simulink model "rover_control"  (R2019b)
settings: Solver=ode3  StartTime=0.0  StopTime=inf  RelTol=1e-3  EnableMultiTasking=on
undefined symbols (not defined in the file or in its folder): Discrete, Time
libraries: embdlinuxlib x13, simulink x3, ctrlSharedLib x2, raspberrypilib x2, sensehatlib x1
(part 2 of 2)

== system rover_control/Plant/Subsystem1/Subsystem1/RGB1 ==
  In1 : Inport
  In2 : Inport  Port=2
  In3 : Inport  Port=3
  B1 : embdlinuxlib/GPIO Write  board=Pi 3 Model B+  gpio=24  direction=Output  blockPlatform=Raspberry Pi
      settings: SourceProductName=Simulink Support Package for Raspberry Pi Hardware  SourceProductBaseCode=RASPPI
  G1 : embdlinuxlib/GPIO Write  board=Pi 3 Model B+  gpio=23  direction=Output  blockPlatform=Raspberry Pi
      settings: SourceProductName=Simulink Support Package for Raspberry Pi Hardware  SourceProductBaseCode=RASPPI
  R1 : embdlinuxlib/GPIO Write  board=Pi 3 Model B+  gpio=22  direction=Output  blockPlatform=Raspberry Pi
      settings: SourceProductName=Simulink Support Package for Raspberry Pi Hardware  SourceProductBaseCode=RASPPI
  wires:
  In1/1 -> R1/1
  In3/1 -> B1/1
  In2/1 -> G1/1

== system rover_control/Plant/Subsystem1/Subsystem1/RGB2 ==
  In1 : Inport
  In2 : Inport  Port=2
  In3 : Inport  Port=3
  B1 : embdlinuxlib/GPIO Write  board=Model B+  gpio=25  direction=Output  blockPlatform=Raspberry Pi
      settings: SourceProductName=Simulink Support Package for Raspberry Pi Hardware  SourceProductBaseCode=RASPPI
  G1 : embdlinuxlib/GPIO Write  board=Model B+  gpio=9  direction=Output  blockPlatform=Raspberry Pi
      settings: SourceProductName=Simulink Support Package for Raspberry Pi Hardware  SourceProductBaseCode=RASPPI
  R1 : embdlinuxlib/GPIO Write  board=Model B+  gpio=10  direction=Output  blockPlatform=Raspberry Pi
      settings: SourceProductName=Simulink Support Package for Raspberry Pi Hardware  SourceProductBaseCode=RASPPI
  wires:
  In2/1 -> G1/1
  In3/1 -> B1/1
  In1/1 -> R1/1

== system rover_control/Plant/Subsystem1/Subsystem1/ServoControl ==
  cam_ud : Inport
  cam_lr : Inport  Port=2
  whl_lr : Inport  Port=3
  Ground : Ground
  MATLAB System : MATLABSystem  System=PCA9685  SlaveAddress=hex2dec('40')  Frequency=60
      mask Type: PCA9685
      mask Display:
      | disp('PCA9685');
      | port_label('input',1,'u1');
      | port_label('input',2,'u2');
      | port_label('input',3,'u3');
      | port_label('input',4,'u4');
      | port_label('input',5,'u5');
      | port_label('input',6,'u6');
      | port_label('input',7,'u7');
      | port_label('input',8,'u8');
      | port_label('input',9,'u9');
      | port_label('input',10,'u10');
      | port_label('input',11,'u11');
      | port_label('input',12,'u12');
  wires:
  Ground/1 -> MATLAB System/11, MATLAB System/12, MATLAB System/10, MATLAB System/4, MATLAB System/5, MATLAB System/6, MATLAB System/7, MATLAB System/8, MATLAB System/9
  cam_lr/1 -> MATLAB System/2
  whl_lr/1 -> MATLAB System/3
  cam_ud/1 -> MATLAB System/1

== system rover_control/Plant/Subsystem2/RPiSystem/RPiSerialSource ==
  Compare To Constant : simulink/Logic and Bit Operations/Compare To Constant  relop===  const=uint8(0)  OutDataTypeStr=boolean
  Constant1 : Constant  Value=zeros(1,164)  OutDataTypeStr=uint8
  Serial Read : raspberrypilib/Serial Read  board=Pi 3 Model B  SCIModule_=/dev/ttyS0  Baudrate_=9600  Parity=None  StopBits_=1  HardwareFlowControl=None  ByteOrder=LittleEndian  DataLength=164  DataType=uint8  OutputStatus=on  SampleTime=0.1  blockPlatform=RaspberryPi
      settings: SourceProductName=Simulink Support Package for Raspberry Pi Hardware  SourceProductBaseCode=RASPPI
  Switch : Switch  Criteria=u2 > Threshold
  gps_vector : Outport
  wires:
  Switch/1 -> gps_vector/1  "gps_vector"
  Serial Read/2 -> Compare To Constant/1
  Constant1/1 -> Switch/3
  Serial Read/1 -> Switch/1  "gps_vector"
  Compare To Constant/1 -> Switch/2

== system rover_control/Plant/Subsystem2/RPiSystem/Tracking3CH ==
  Bus Creator : BusCreator  Inputs=3
  C : embdlinuxlib/GPIO Read  board=Pi 3 Model B+  gpio=16  internalResistor=Off  sampleTime=0.1  direction=Input  blockPlatform=Raspberry Pi
      settings: SourceProductName=Simulink Support Package for Raspberry Pi Hardware  SourceProductBaseCode=RASPPI
  Display : Display
  Display1 : Display
  Display2 : Display
  L : embdlinuxlib/GPIO Read  board=Pi 3 Model B+  gpio=19  internalResistor=Off  sampleTime=0.1  direction=Input  blockPlatform=Raspberry Pi
      settings: SourceProductName=Simulink Support Package for Raspberry Pi Hardware  SourceProductBaseCode=RASPPI
  NOT : Logic  Operator=NOT  IconShape=distinctive  AllPortsSameDT=off  OutDataTypeStr=boolean
  NOT1 : Logic  Operator=NOT  IconShape=distinctive  AllPortsSameDT=off  OutDataTypeStr=boolean
  NOT2 : Logic  Operator=NOT  IconShape=distinctive  AllPortsSameDT=off  OutDataTypeStr=boolean
  R : embdlinuxlib/GPIO Read  board=Pi 3 Model B+  gpio=20  internalResistor=Off  sampleTime=0.1  direction=Input  blockPlatform=Raspberry Pi
      settings: SourceProductName=Simulink Support Package for Raspberry Pi Hardware  SourceProductBaseCode=RASPPI
  tracking : Outport
  wires:
  Bus Creator/1 -> tracking/1
  L/1 -> NOT/1
  C/1 -> NOT1/1
  R/1 -> NOT2/1
  NOT/1 -> Display/1, Bus Creator/1  "leftLineDetected"
  NOT1/1 -> Display1/1, Bus Creator/2  "centerLineDetected"
  NOT2/1 -> Display2/1, Bus Creator/3  "rightLineDetected"

== system rover_control/Plant/Subsystem2/RPiSystem/UltrasonicSensor ==
  MATLAB System : MATLABSystem  System=UltrasonicRead  EchoPinNumber=echo_gpio  TriggerPinNumber=trigger_gpio  SampleTime=sampleTime
      mask Type: UltrasonicRead
      mask Display:
      | disp('Ultrasonic Read');
      | port_label('output',1,'y');
  Out1 : Outport  VectorParamsAs1DForOutWhenUnconnected=off
  wires:
  MATLAB System/1 -> Out1/1

== system rover_control/Controller/Subsystem/GPS/CharacterBufferLoad/NMEASentenceExtract ==
  serial_vector : Inport
  ASCII to String : ASCIIToString
  MATLAB Function : MATLAB Function  TreatAsAtomicUnit=on
  string : Outport
  wires:
  serial_vector/1 -> MATLAB Function/1(u)
  ASCII to String/1 -> string/1
  MATLAB Function/1(y) -> ASCII to String/1

== system rover_control/Controller/Subsystem/GPS/GGA Decoder/Subsystem ==
  In1 : Inport
  Constant : Constant  OutDataTypeStr=uint8
  Constant1 : Constant  Value=2  OutDataTypeStr=uint8
  Constant2 : Constant  Value=3  OutDataTypeStr=uint8
  Constant4 : Constant  Value=5  OutDataTypeStr=uint8
  String Concatenate : StringConcatenate  Inputs=5
  String Constant : StringConstant  String="\":\""
  Substring : Substring
  Substring1 : Substring
  Substring2 : Substring
  Out1 : Outport  VectorParamsAs1DForOutWhenUnconnected=off
  wires:
  Constant/1 -> Substring/2
  Constant2/1 -> Substring1/2
  Constant4/1 -> Substring2/2
  In1/1 -> Substring2/1, Substring/1, Substring1/1
  Constant1/1 -> Substring2/3, Substring1/3, Substring/3
  Substring1/1 -> String Concatenate/3
  Substring/1 -> String Concatenate/1
  Substring2/1 -> String Concatenate/5
  String Constant/1 -> String Concatenate/4, String Concatenate/2
  String Concatenate/1 -> Out1/1

== system rover_control/Controller/Subsystem/GPS/GLL Decoder/Subsystem ==
  In1 : Inport
  Constant : Constant  OutDataTypeStr=uint8
  Constant1 : Constant  Value=2  OutDataTypeStr=uint8
  Constant2 : Constant  Value=3  OutDataTypeStr=uint8
  Constant4 : Constant  Value=5  OutDataTypeStr=uint8
  String Concatenate : StringConcatenate  Inputs=5
  String Constant : StringConstant  String="\":\""
  Substring : Substring
  Substring1 : Substring
  Substring2 : Substring
  Out1 : Outport  VectorParamsAs1DForOutWhenUnconnected=off
  wires:
  String Concatenate/1 -> Out1/1
  String Constant/1 -> String Concatenate/2, String Concatenate/4
  Substring2/1 -> String Concatenate/5
  Substring/1 -> String Concatenate/1
  Substring1/1 -> String Concatenate/3
  Constant1/1 -> Substring/3, Substring1/3, Substring2/3
  In1/1 -> Substring1/1, Substring/1, Substring2/1
  Constant4/1 -> Substring2/2
  Constant2/1 -> Substring1/2
  Constant/1 -> Substring/2

== system rover_control/Controller/Subsystem/GPS/GSA Decoder/Subsystem ==
  In1 : Inport
  ASCII to String : ASCIIToString
  ASCII to String1 : ASCIIToString
  MATLAB Function : MATLAB Function  TreatAsAtomicUnit=on
  Scan String : ScanString  Format="\"%hu,%hu,%hu,%hu,%hu,%hu,%hu,%hu,%hu,%hu,%hu,%hu\""
  String to ASCII : StringToASCII  OutputVectorSize=80
  Vector Concatenate : Concatenate  NumInputs=12
  prns : Outport
  rem : Outport  Port=2
  wires:
  In1/1 -> String to ASCII/1
  String to ASCII/1 -> MATLAB Function/1(u)
  MATLAB Function/2(prns) -> ASCII to String1/1
  MATLAB Function/1(y) -> ASCII to String/1
  ASCII to String/1 -> rem/1
  ASCII to String1/1 -> Scan String/1
  Scan String/1 -> Vector Concatenate/1
  Scan String/2 -> Vector Concatenate/2
  Scan String/3 -> Vector Concatenate/3
  Scan String/4 -> Vector Concatenate/4
  Scan String/5 -> Vector Concatenate/5
  Scan String/6 -> Vector Concatenate/6
  Scan String/7 -> Vector Concatenate/7
  Scan String/8 -> Vector Concatenate/8
  Scan String/9 -> Vector Concatenate/9
  Scan String/10 -> Vector Concatenate/10
  Scan String/11 -> Vector Concatenate/11
  Scan String/12 -> Vector Concatenate/12
  Vector Concatenate/1 -> prns/1

== system rover_control/Controller/Subsystem/GPS/RMC Decoder/Subsystem ==
  In1 : Inport
  Constant : Constant  OutDataTypeStr=uint8
  Constant1 : Constant  Value=2  OutDataTypeStr=uint8
  Constant2 : Constant  Value=3  OutDataTypeStr=uint8
  Constant4 : Constant  Value=5  OutDataTypeStr=uint8
  String Concatenate : StringConcatenate  Inputs=5
  String Constant : StringConstant  String="\":\""
  Substring : Substring
  Substring1 : Substring
  Substring2 : Substring
  Out1 : Outport  VectorParamsAs1DForOutWhenUnconnected=off
  wires:
  Constant/1 -> Substring/2
  Constant2/1 -> Substring1/2
  Constant4/1 -> Substring2/2
  In1/1 -> Substring2/1, Substring/1, Substring1/1
  Constant1/1 -> Substring2/3, Substring1/3, Substring/3
  Substring1/1 -> String Concatenate/3
  Substring/1 -> String Concatenate/1
  Substring2/1 -> String Concatenate/5
  String Constant/1 -> String Concatenate/4, String Concatenate/2
  String Concatenate/1 -> Out1/1

== system rover_control/Controller/Subsystem/GPS/RMC Decoder/Subsystem1 ==
  In1 : Inport
  Constant : Constant  Value=3  OutDataTypeStr=uint8
  Constant1 : Constant  Value=2  OutDataTypeStr=uint8
  Constant2 : Constant  OutDataTypeStr=uint8
  Constant4 : Constant  Value=5  OutDataTypeStr=uint8
  String Concatenate : StringConcatenate  Inputs=5
  String Constant : StringConstant  String="\"/\""
  Substring : Substring
  Substring1 : Substring
  Substring2 : Substring
  Out1 : Outport  VectorParamsAs1DForOutWhenUnconnected=off
  wires:
  Constant/1 -> Substring/2
  Constant2/1 -> Substring1/2
  Constant4/1 -> Substring2/2
  In1/1 -> Substring2/1, Substring/1, Substring1/1
  Constant1/1 -> Substring2/3, Substring1/3, Substring/3
  Substring1/1 -> String Concatenate/3
  Substring/1 -> String Concatenate/1
  Substring2/1 -> String Concatenate/5
  String Constant/1 -> String Concatenate/4, String Concatenate/2
  String Concatenate/1 -> Out1/1

== matlab function rover_control/Controller/Subsystem/GPS/GSA Decoder/Subsystem/MATLAB Function ==
  data: y output; u input; prns output
function [y, prns] = gsa(u)
%UNTITLED Summary of this function goes here
%   Detailed explanation goes here
y = zeros(size(u),'uint8');
num_prns = 12;
prns = zeros(size(u),'uint8');
idx = find(u == hex2dec('2c')) ;
% prns = zeros(1,12,'uint16');
%A,3,66,84,74,75,76,85,,,,,,,1.47,0.78,1.24,*17

sIdx = 1;
% for i = 1:length(prns)
%     new_string = u(sIdx:idx(i)-1);
%     if (~isempty(new_string))
%         prns(i) = uint16(str2double(new_string));
%     end
%     sIdx = idx(i)+1;
% end
for i=1:num_prns
    %66,34,23,53,,,,,,,,,,
    new_string = u(sIdx:idx(i)-1);
    if (~isempty(new_string))
        prns(sIdx:sIdx+length(new_string)) = [new_string, ','];
        z = length(new_string);
    else
        if (i == num_prns)
            prns(sIdx) = '0';
            z = 1;
        else
            prns(sIdx:sIdx+1) = '0,';
            z = 1;
        end
    end
%     prns(pIdx:idx(i)) = u(sIdx:idx(i));
    sIdx = sIdx + z + 1;
%     disp(i)
%     disp(char(prns))
end
y(1:length(u)-idx(12)) = u(idx(12)+1:end);
% pdop = str2double(char(u(sIdx:
% hdop = 
% vdop = 
% checksum = 
end
% function [y, prns] = gsa_u(u)
% y = zeros(1,80,'uint8');
% [z,prns] = gsa(u);
% y(1:length(z)) = z;
% end

== matlab function rover_control/Controller/Subsystem/GPS/CharacterBufferLoad/NMEASentenceExtract/MATLAB Function ==
  data: u input; y output size=[1 80]
function y  = gps_data_handle(u)
persistent start;
persistent new_input;
persistent prev_u;
% \r - 0xD (carriage return) \n - 0xA )(line feed)
% 
% d = find(u == hex2dec('d'));
% r = find(u == hex2dec('a'));
%
% $ - decimal 36 hex 0x24
if (isempty(start))
    start = false;
    new_input = zeros(1,length(u)*2,'like',u);
    prev_u = zeros(size(u),'like',u);
end
if (~start)
    start = true;
    prev_u = u;
    % check if data is complete
    if (u(1) ~= hex2dec('24'))
        % find first index that has '$'
        idx = find(u,1,'first');
%         z = zeros(size(u));
        u = shift_vector(u, idx(1)-1);
    end
    new_input(1:length(u)) = u;
end
        
if (~isequal(u,prev_u))
    idx = find(new_input == 0,1,'first');
    new_input(idx(1):idx(1)+length(u)-1) = u(1:end);
    prev_u = u;
end

sentence = zeros(1,80, 'like',u);
idx = find(new_input == hex2dec('24'), 2, 'first');
if (length(idx) == 2)
    % this is needed if the carriage return and line feed get treated as
    % separate characters like it does in raspberry pi serial block
    crlf = 2;
    sentence(1:idx(2)-idx(1)-crlf) = new_input(idx(1):idx(2)-1-crlf);
    new_input = shift_vector(new_input, idx(2)-1);
end

y = sentence;
end

function y = shift_vector(u, K)
 
y=zeros(size(u),'like',u);
% n=2; %Shift units
y(1:end-K+1)=u(K:end);
end

== matlab function rover_control/Controller/Subsystem/GPS/VTG Decoder/MATLAB Function ==
  data: u input; ttrack output; mtrack output; gs_k output; gs_kph output; sig_ent output; checksum output
function [ttrack,mtrack,gs_k,gs_kph,sig_ent,checksum] = vtg(u)
%,T,,M,0.346,N,0.642,K,A*3C
ttrack = zeros(1,8,'uint8');
mtrack = zeros(1,8,'uint8');
gs_k = zeros(1,8,'uint8');
gs_kph = zeros(1,8,'uint8');
sig_ent = zeros(1,1, 'uint8');
checksum = zeros(1,2, 'uint8');
idx = find(u == hex2dec('2c')) ;
if (idx(1) > 1)
    ttrack(1:idx(1)-1) = u(1:idx(1)-1);
%     ttrack(1) = sscanf(u(1:idx(1)-1), '%lf');
%     ttrack(1) = str2double(u(1:idx(1)-1));
end
if (idx(3)- idx(2) > 1)
    mtrack(1:idx(3) - idx(2)) = u(idx(2)+1:idx(3)-1);
%     mtrack(1) = str2double(u(idx(2)+1:idx(3)-1));
end
if (idx(5)-idx(4) > 1)
    gs_k(1:idx(5)-idx(4)) = u(idx(4)+1:idx(5)-1);
%     gs_k(1) = str2double(u(idx(4)+1:idx(5)-1));
end
if (idx(7)-idx(6) > 1)
    gs_kph(1:idx(7)-idx(6)) = u(idx(6)+1:idx(7)-1);
%     gs_kph(1) = str2double(u(idx(6)+1:idx(7)-1));
end
sig_ent(1) = u(idx(8)+1);
checksum(1:end) = u(idx(8)+3:end);
end

== matlab function rover_control/Controller/Subsystem/GPS/RMC Decoder/MATLAB Function ==
  data: u input; y output
function y = rmc(u)
% example string
%220725.00,A,4349.94607,N,09643.86727,W,0.669,,021219,,,A*7E
idx = find(u == hex2dec('2c'));
pos = diff(idx);
pos = [idx(1) pos length(u)-idx(end)];

y = zeros(1,80,'uint8');
yIdx=1;
uIdx=1;
for i=1:length(pos)
    if (pos(i) == 1)
        y(yIdx:yIdx+1) = ['0' ','];
        yIdx = yIdx + 2;
        uIdx = idx(i)+1;
    else
        y(yIdx:yIdx+pos(i)-1) = u(uIdx:uIdx+pos(i)-1);
        yIdx = yIdx + pos(i);
        uIdx = uIdx + pos(i);
    end
end

== stateflow chart rover_control/Plant/Subsystem1/Subsystem1/MotorDrive/Chart ==
  (default) -> (junction 14) : % Direction logic
  (junction 14) -> (junction 15) [order 1] : [direction > 0]
  (junction 14) -> (junction 16) [order 2]
  (junction 15) -> (junction 20) : {fwd = true;
      |  rev=false;}
  (junction 16) -> (junction 17) [order 1] : [direction < 0]
  (junction 16) -> (junction 18) [order 2] : {fwd=false;
      | rev=false;}
  (junction 17) -> (junction 19) : {fwd=false;
      | rev=true;}
  (junction 19) -> (junction 18)
  (junction 20) -> (junction 19)
  (junction 18) -> (junction 21)
  data: fwd output; rev output; direction input

== stateflow chart rover_control/Controller/CollisionAvoidance/Chart ==
  data: data input

== stateflow chart rover_control/Controller/Subsystem/Chart ==
  data: gga input; data output
